simulink model "UserTire"  (Simulink 7.9)
settings: Solver=ode45  StartTime=0.0  StopTime=inf  RelTol=1e-3
PreLoadFcn:
  | UserTire_params
undefined symbols (not defined in the file): FricCoeff, Longitudinal, Side
libraries: simulink x1, CarMaker4SL x1
(part 2 of 2)

== system UserTire/CarMaker/IPG Vehicle/CarAndTrailer/Trailer/CreateBus Vhcl.Wheel.RL ==
  In1 : Inport
  Bus Creator3 : BusCreator  Inputs=14
  Demux3 : Demux  Outputs=14
  Out1 : Outport
  wires:
  Demux3/14 -> Bus Creator3/14  "Vhcl Wheel RL Trq_WhlBearing"
  Demux3/13 -> Bus Creator3/13  "Vhcl Wheel RL Trq_T2W"
  Demux3/12 -> Bus Creator3/12  "Vhcl Wheel RL SideSlip"
  Demux3/11 -> Bus Creator3/11  "Vhcl Wheel RL LongSlip"
  Demux3/10 -> Bus Creator3/10  "Vhcl Wheel RL vBelt"
  Demux3/9 -> Bus Creator3/9  "Vhcl Wheel RL Fz"
  Demux3/8 -> Bus Creator3/8  "Vhcl Wheel RL Fy"
  Demux3/7 -> Bus Creator3/7  "Vhcl Wheel RL Fx"
  Demux3/6 -> Bus Creator3/6  "Vhcl Wheel RL r_zxy z"
  Demux3/5 -> Bus Creator3/5  "Vhcl Wheel RL r_zxy y"
  Demux3/4 -> Bus Creator3/4  "Vhcl Wheel RL r_zxy x"
  Demux3/3 -> Bus Creator3/3  "Vhcl Wheel RL t z"
  Demux3/2 -> Bus Creator3/2  "Vhcl Wheel RL t y"
  In1/1 -> Demux3/1
  Bus Creator3/1 -> Out1/1
  Demux3/1 -> Bus Creator3/1  "Vhcl Wheel RL t x"

== system UserTire/CarMaker/IPG Vehicle/CarAndTrailer/Trailer/CreateBus Vhcl.Wheel.RR ==
  In1 : Inport
  Bus Creator3 : BusCreator  Inputs=14
  Demux3 : Demux  Outputs=14
  Out1 : Outport
  wires:
  Demux3/14 -> Bus Creator3/14  "Vhcl Wheel RR Trq_WhlBearing"
  Demux3/13 -> Bus Creator3/13  "Vhcl Wheel RR Trq_T2W"
  Demux3/12 -> Bus Creator3/12  "Vhcl Wheel RR SideSlip"
  Demux3/11 -> Bus Creator3/11  "Vhcl Wheel RR LongSlip"
  Demux3/10 -> Bus Creator3/10  "Vhcl Wheel RR vBelt"
  Demux3/9 -> Bus Creator3/9  "Vhcl Wheel RR Fz"
  Demux3/8 -> Bus Creator3/8  "Vhcl Wheel RR Fy"
  Demux3/7 -> Bus Creator3/7  "Vhcl Wheel RR Fx"
  Demux3/6 -> Bus Creator3/6  "Vhcl Wheel RR r_zxy z"
  Demux3/5 -> Bus Creator3/5  "Vhcl Wheel RR r_zxy y"
  Demux3/4 -> Bus Creator3/4  "Vhcl Wheel RR r_zxy x"
  Demux3/3 -> Bus Creator3/3  "Vhcl Wheel RR t z"
  Demux3/2 -> Bus Creator3/2  "Vhcl Wheel RR t y"
  In1/1 -> Demux3/1
  Bus Creator3/1 -> Out1/1
  Demux3/1 -> Bus Creator3/1  "Vhcl Wheel RR t x"

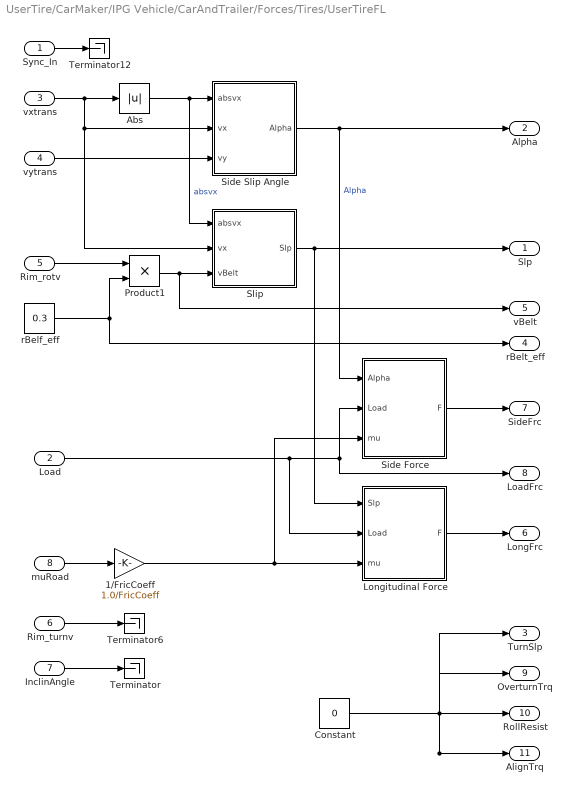
== system UserTire/CarMaker/IPG Vehicle/CarAndTrailer/Forces/Tires/UserTireFL ==
  Sync_In : Inport
  Load : Inport  Port=2
  vxtrans : Inport  Port=3
  vytrans : Inport  Port=4
  Rim_rotv : Inport  Port=5
  Rim_turnv : Inport  Port=6
  InclinAngle : Inport  Port=7
  muRoad : Inport  Port=8
  1/FricCoeff : Gain  Gain=1.0/FricCoeff  SaturateOnIntegerOverflow=on  OutDataTypeStr=Inherit: Same as input  ParamDataTypeStr=Inherit: Same as input
  Abs : Abs  SaturateOnIntegerOverflow=on
  Constant : Constant  Value=0
  Longitudinal Force : Subsystem
  Product1 : Product  Inputs=**  SaturateOnIntegerOverflow=on  InputSameDT=on  OutDataTypeStr=Inherit: Same as first input
  Side Force : Subsystem
  Side Slip Angle : Subsystem
  Slip : Subsystem
  Terminator : Terminator
  Terminator12 : Terminator
  Terminator6 : Terminator
  rBelf_eff : Constant  Value=0.3
  Slp : Outport
  Alpha : Outport  Port=2
  TurnSlp : Outport  Port=3
  rBelt_eff : Outport  Port=4
  vBelt : Outport  Port=5
  LongFrc : Outport  Port=6
  SideFrc : Outport  Port=7
  LoadFrc : Outport  Port=8
  OverturnTrq : Outport  Port=9
  RollResist : Outport  Port=10
  AlignTrq : Outport  Port=11
  wires:
  1/FricCoeff/1 -> Side Force/3(mu), Longitudinal Force/3(mu)
  muRoad/1 -> 1/FricCoeff/1
  Side Force/1(F) -> SideFrc/1
  Constant/1 -> OverturnTrq/1, RollResist/1, AlignTrq/1, TurnSlp/1
  InclinAngle/1 -> Terminator/1
  Longitudinal Force/1(F) -> LongFrc/1
  Load/1 -> LoadFrc/1, Side Force/2(Load), Longitudinal Force/2(Load)
  Slip/1(Slp) -> Slp/1, Longitudinal Force/1(Slp)
  Side Slip Angle/1(Alpha) -> Alpha/1, Side Force/1(Alpha)  "Alpha"
  Abs/1 -> Slip/1(absvx), Side Slip Angle/1(absvx)  "absvx"
  vytrans/1 -> Side Slip Angle/3(vy)
  vxtrans/1 -> Slip/2(vx), Side Slip Angle/2(vx), Abs/1
  Sync_In/1 -> Terminator12/1
  Rim_turnv/1 -> Terminator6/1
  Rim_rotv/1 -> Product1/1
  Product1/1 -> Slip/3(vBelt), vBelt/1
  rBelf_eff/1 -> Product1/2, rBelt_eff/1

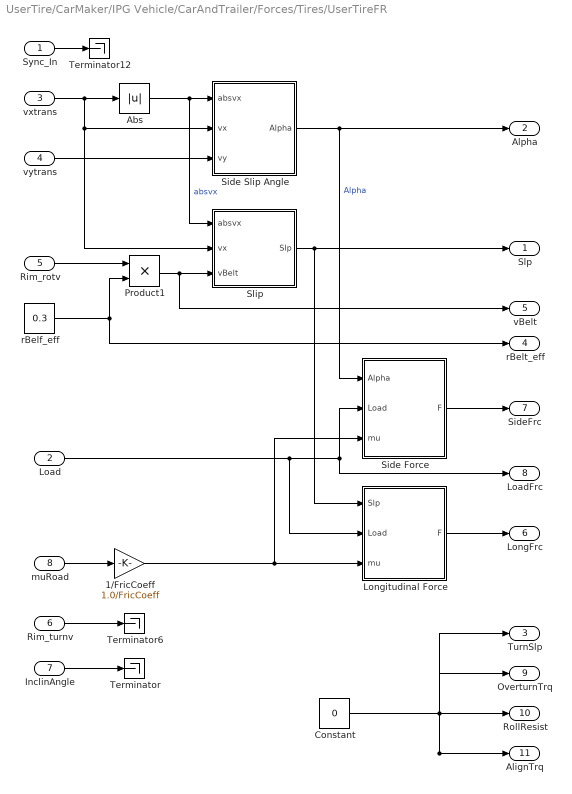
== system UserTire/CarMaker/IPG Vehicle/CarAndTrailer/Forces/Tires/UserTireFR ==
  Sync_In : Inport
  Load : Inport  Port=2
  vxtrans : Inport  Port=3
  vytrans : Inport  Port=4
  Rim_rotv : Inport  Port=5
  Rim_turnv : Inport  Port=6
  InclinAngle : Inport  Port=7
  muRoad : Inport  Port=8
  1/FricCoeff : Gain  Gain=1.0/FricCoeff  SaturateOnIntegerOverflow=on  OutDataTypeStr=Inherit: Same as input  ParamDataTypeStr=Inherit: Same as input
  Abs : Abs  SaturateOnIntegerOverflow=on
  Constant : Constant  Value=0
  Longitudinal Force : Subsystem
  Product1 : Product  Inputs=**  SaturateOnIntegerOverflow=on  InputSameDT=on  OutDataTypeStr=Inherit: Same as first input
  Side Force : Subsystem
  Side Slip Angle : Subsystem
  Slip : Subsystem
  Terminator : Terminator
  Terminator12 : Terminator
  Terminator6 : Terminator
  rBelf_eff : Constant  Value=0.3
  Slp : Outport
  Alpha : Outport  Port=2
  TurnSlp : Outport  Port=3
  rBelt_eff : Outport  Port=4
  vBelt : Outport  Port=5
  LongFrc : Outport  Port=6
  SideFrc : Outport  Port=7
  LoadFrc : Outport  Port=8
  OverturnTrq : Outport  Port=9
  RollResist : Outport  Port=10
  AlignTrq : Outport  Port=11
  wires:
  1/FricCoeff/1 -> Side Force/3(mu), Longitudinal Force/3(mu)
  muRoad/1 -> 1/FricCoeff/1
  Side Force/1(F) -> SideFrc/1
  Constant/1 -> OverturnTrq/1, RollResist/1, AlignTrq/1, TurnSlp/1
  InclinAngle/1 -> Terminator/1
  Longitudinal Force/1(F) -> LongFrc/1
  Load/1 -> LoadFrc/1, Side Force/2(Load), Longitudinal Force/2(Load)
  Slip/1(Slp) -> Slp/1, Longitudinal Force/1(Slp)
  Side Slip Angle/1(Alpha) -> Alpha/1, Side Force/1(Alpha)  "Alpha"
  Abs/1 -> Slip/1(absvx), Side Slip Angle/1(absvx)  "absvx"
  vytrans/1 -> Side Slip Angle/3(vy)
  vxtrans/1 -> Slip/2(vx), Side Slip Angle/2(vx), Abs/1
  Sync_In/1 -> Terminator12/1
  Rim_turnv/1 -> Terminator6/1
  Rim_rotv/1 -> Product1/1
  Product1/1 -> Slip/3(vBelt), vBelt/1
  rBelf_eff/1 -> Product1/2, rBelt_eff/1

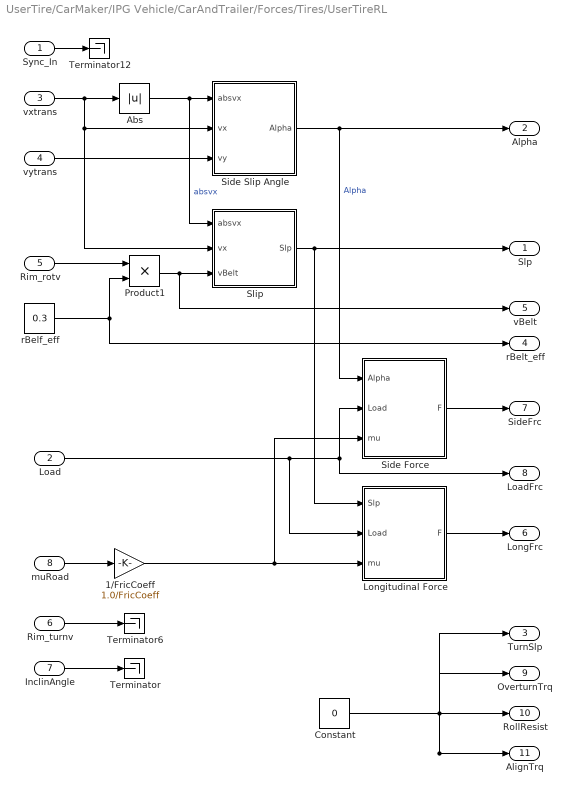
== system UserTire/CarMaker/IPG Vehicle/CarAndTrailer/Forces/Tires/UserTireRL ==
  Sync_In : Inport
  Load : Inport  Port=2
  vxtrans : Inport  Port=3
  vytrans : Inport  Port=4
  Rim_rotv : Inport  Port=5
  Rim_turnv : Inport  Port=6
  InclinAngle : Inport  Port=7
  muRoad : Inport  Port=8
  1/FricCoeff : Gain  Gain=1.0/FricCoeff  SaturateOnIntegerOverflow=on  OutDataTypeStr=Inherit: Same as input  ParamDataTypeStr=Inherit: Same as input
  Abs : Abs  SaturateOnIntegerOverflow=on
  Constant : Constant  Value=0
  Longitudinal Force : Subsystem
  Product1 : Product  Inputs=**  SaturateOnIntegerOverflow=on  InputSameDT=on  OutDataTypeStr=Inherit: Same as first input
  Side Force : Subsystem
  Side Slip Angle : Subsystem
  Slip : Subsystem
  Terminator : Terminator
  Terminator12 : Terminator
  Terminator6 : Terminator
  rBelf_eff : Constant  Value=0.3
  Slp : Outport
  Alpha : Outport  Port=2
  TurnSlp : Outport  Port=3
  rBelt_eff : Outport  Port=4
  vBelt : Outport  Port=5
  LongFrc : Outport  Port=6
  SideFrc : Outport  Port=7
  LoadFrc : Outport  Port=8
  OverturnTrq : Outport  Port=9
  RollResist : Outport  Port=10
  AlignTrq : Outport  Port=11
  wires:
  1/FricCoeff/1 -> Side Force/3(mu), Longitudinal Force/3(mu)
  muRoad/1 -> 1/FricCoeff/1
  Side Force/1(F) -> SideFrc/1
  Constant/1 -> OverturnTrq/1, RollResist/1, AlignTrq/1, TurnSlp/1
  InclinAngle/1 -> Terminator/1
  Longitudinal Force/1(F) -> LongFrc/1
  Load/1 -> LoadFrc/1, Side Force/2(Load), Longitudinal Force/2(Load)
  Slip/1(Slp) -> Slp/1, Longitudinal Force/1(Slp)
  Side Slip Angle/1(Alpha) -> Alpha/1, Side Force/1(Alpha)  "Alpha"
  Abs/1 -> Slip/1(absvx), Side Slip Angle/1(absvx)  "absvx"
  vytrans/1 -> Side Slip Angle/3(vy)
  vxtrans/1 -> Slip/2(vx), Side Slip Angle/2(vx), Abs/1
  Sync_In/1 -> Terminator12/1
  Rim_turnv/1 -> Terminator6/1
  Rim_rotv/1 -> Product1/1
  Product1/1 -> Slip/3(vBelt), vBelt/1
  rBelf_eff/1 -> Product1/2, rBelt_eff/1

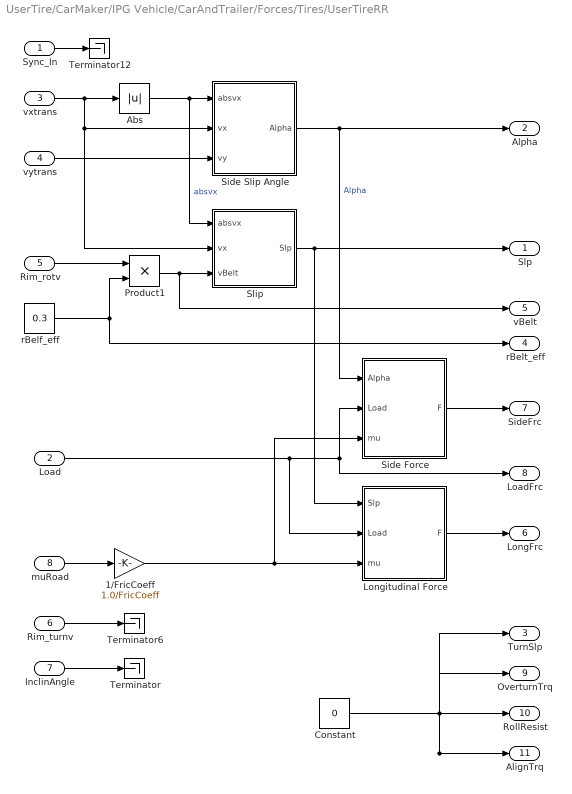
== system UserTire/CarMaker/IPG Vehicle/CarAndTrailer/Forces/Tires/UserTireRR ==
  Sync_In : Inport
  Load : Inport  Port=2
  vxtrans : Inport  Port=3
  vytrans : Inport  Port=4
  Rim_rotv : Inport  Port=5
  Rim_turnv : Inport  Port=6
  InclinAngle : Inport  Port=7
  muRoad : Inport  Port=8
  1/FricCoeff : Gain  Gain=1.0/FricCoeff  SaturateOnIntegerOverflow=on  OutDataTypeStr=Inherit: Same as input  ParamDataTypeStr=Inherit: Same as input
  Abs : Abs  SaturateOnIntegerOverflow=on
  Constant : Constant  Value=0
  Longitudinal Force : Subsystem
  Product1 : Product  Inputs=**  SaturateOnIntegerOverflow=on  InputSameDT=on  OutDataTypeStr=Inherit: Same as first input
  Side Force : Subsystem
  Side Slip Angle : Subsystem
  Slip : Subsystem
  Terminator : Terminator
  Terminator12 : Terminator
  Terminator6 : Terminator
  rBelf_eff : Constant  Value=0.3
  Slp : Outport
  Alpha : Outport  Port=2
  TurnSlp : Outport  Port=3
  rBelt_eff : Outport  Port=4
  vBelt : Outport  Port=5
  LongFrc : Outport  Port=6
  SideFrc : Outport  Port=7
  LoadFrc : Outport  Port=8
  OverturnTrq : Outport  Port=9
  RollResist : Outport  Port=10
  AlignTrq : Outport  Port=11
  wires:
  1/FricCoeff/1 -> Side Force/3(mu), Longitudinal Force/3(mu)
  muRoad/1 -> 1/FricCoeff/1
  Side Force/1(F) -> SideFrc/1
  Constant/1 -> OverturnTrq/1, RollResist/1, AlignTrq/1, TurnSlp/1
  InclinAngle/1 -> Terminator/1
  Longitudinal Force/1(F) -> LongFrc/1
  Load/1 -> LoadFrc/1, Side Force/2(Load), Longitudinal Force/2(Load)
  Slip/1(Slp) -> Slp/1, Longitudinal Force/1(Slp)
  Side Slip Angle/1(Alpha) -> Alpha/1, Side Force/1(Alpha)  "Alpha"
  Abs/1 -> Slip/1(absvx), Side Slip Angle/1(absvx)  "absvx"
  vytrans/1 -> Side Slip Angle/3(vy)
  vxtrans/1 -> Slip/2(vx), Side Slip Angle/2(vx), Abs/1
  Sync_In/1 -> Terminator12/1
  Rim_turnv/1 -> Terminator6/1
  Rim_rotv/1 -> Product1/1
  Product1/1 -> Slip/3(vBelt), vBelt/1
  rBelf_eff/1 -> Product1/2, rBelt_eff/1

== system UserTire/CarMaker/IPG Vehicle/CarAndTrailer/Forces/Tires/UserTireFL/Longitudinal Force ==
  Slp : Inport
  Load : Inport  Port=2
  mu : Inport  Port=3
  Abs2 : Abs  SaturateOnIntegerOverflow=on
  Longitudinal ForceRate : Constant  Value=Longitudinal.ForceRate
  Longitudinal FrictionRate : Constant  Value=Longitudinal.FrictionRate
  Product1 : Product  SaturateOnIntegerOverflow=on  InputSameDT=on  OutDataTypeStr=Inherit: Same as first input
  Product3 : Product  Inputs=3  SaturateOnIntegerOverflow=on  InputSameDT=on  OutDataTypeStr=Inherit: Same as first input
  Product4 : Product  SaturateOnIntegerOverflow=on  InputSameDT=on  OutDataTypeStr=Inherit: Same as first input
  Product5 : Product  SaturateOnIntegerOverflow=on  InputSameDT=on  OutDataTypeStr=Inherit: Same as first input
  Relational Operator1 : RelationalOperator  Operator=>  InputSameDT=on
  Sign : Signum
  Switch1 : Switch  Threshold=1  SaturateOnIntegerOverflow=on  InputSameDT=on
  F : Outport
  wires:
  mu/1 -> Product1/2
  Product1/1 -> F/1
  Switch1/1 -> Product1/1
  Load/1 -> Product4/1, Product3/2
  Slp/1 -> Product3/1
  Sign/1 -> Product5/1
  Product5/1 -> Switch1/1
  Relational Operator1/1 -> Switch1/2
  Abs2/1 -> Relational Operator1/1  "absF"
  Product4/1 -> Product5/2, Relational Operator1/2  "d"
  Product3/1 -> Switch1/3, Abs2/1, Sign/1  "F"
  Longitudinal FrictionRate/1 -> Product4/2
  Longitudinal ForceRate/1 -> Product3/3

== system UserTire/CarMaker/IPG Vehicle/CarAndTrailer/Forces/Tires/UserTireFL/Side Force ==
  Alpha : Inport
  Load : Inport  Port=2
  mu : Inport  Port=3
  -Side ForceAmplify : Constant  Value=-Side.ForceAmplify
  Abs2 : Abs  SaturateOnIntegerOverflow=on
  Product : Product  Inputs=3  SaturateOnIntegerOverflow=on  InputSameDT=on  OutDataTypeStr=Inherit: Same as first input
  Product3 : Product  Inputs=3  SaturateOnIntegerOverflow=on  InputSameDT=on  OutDataTypeStr=Inherit: Same as first input
  Product4 : Product  SaturateOnIntegerOverflow=on  InputSameDT=on  OutDataTypeStr=Inherit: Same as first input
  Product5 : Product  SaturateOnIntegerOverflow=on  InputSameDT=on  OutDataTypeStr=Inherit: Same as first input
  Relational Operator1 : RelationalOperator  Operator=>  InputSameDT=on
  Side ForceRate : Constant  Value=Side.ForceRate
  Side FrictionRate : Constant  Value=Side.FrictionRate
  Sign : Signum
  Switch1 : Switch  Threshold=1  SaturateOnIntegerOverflow=on  InputSameDT=on
  F : Outport
  wires:
  mu/1 -> Product/3
  -Side ForceAmplify/1 -> Product/1
  Product/1 -> F/1
  Switch1/1 -> Product/2
  Load/1 -> Product4/1, Product3/2
  Alpha/1 -> Product3/1
  Sign/1 -> Product5/1
  Product5/1 -> Switch1/1
  Relational Operator1/1 -> Switch1/2
  Abs2/1 -> Relational Operator1/1  "absF"
  Product4/1 -> Product5/2, Relational Operator1/2  "d"
  Product3/1 -> Switch1/3, Abs2/1, Sign/1  "F"
  Side FrictionRate/1 -> Product4/2
  Side ForceRate/1 -> Product3/3

== system UserTire/CarMaker/IPG Vehicle/CarAndTrailer/Forces/Tires/UserTireFL/Side Slip Angle ==
  absvx : Inport
  vx : Inport  Port=2
  vy : Inport  Port=3
  Constant6 : Constant  Value=0.25
  Constant7 : Constant  Value=0
  Relational Operator3 : RelationalOperator  Operator=>  InputSameDT=on
  Switch3 : Switch  Threshold=1  SaturateOnIntegerOverflow=on  InputSameDT=on
  Trigonometric Function1 : Trigonometry  Operator=atan2
  Alpha : Outport
  wires:
  Constant7/1 -> Switch3/3
  Trigonometric Function1/1 -> Switch3/1
  vy/1 -> Trigonometric Function1/1
  vx/1 -> Trigonometric Function1/2
  Switch3/1 -> Alpha/1
  absvx/1 -> Relational Operator3/1
  Relational Operator3/1 -> Switch3/2
  Constant6/1 -> Relational Operator3/2

== system UserTire/CarMaker/IPG Vehicle/CarAndTrailer/Forces/Tires/UserTireFL/Slip ==
  absvx : Inport
  vx : Inport  Port=2
  vBelt : Inport  Port=3
  Abs2 : Abs  SaturateOnIntegerOverflow=on
  Constant1 : Constant  Value=0
  Constant3 : Constant  Value=0
  Constant4 : Constant  Value=0.000001
  Product1 : Product  Inputs=*/  SaturateOnIntegerOverflow=on  InputSameDT=on  OutDataTypeStr=Inherit: Same as first input
  Relational Operator1 : RelationalOperator  Operator===  InputSameDT=on
  Relational Operator3 : RelationalOperator  Operator=<  InputSameDT=on
  Sum1 : Sum  Inputs=-+  SaturateOnIntegerOverflow=on  InputSameDT=on  OutDataTypeStr=Inherit: Same as first input
  Switch1 : Switch  Threshold=1  SaturateOnIntegerOverflow=on  InputSameDT=on
  Switch3 : Switch  Threshold=1  SaturateOnIntegerOverflow=on  InputSameDT=on
  Slp : Outport
  wires:
  Product1/1 -> Slp/1
  Constant4/1 -> Switch1/1
  Switch1/1 -> Product1/2  "not zero"
  Constant3/1 -> Relational Operator1/1
  Relational Operator1/1 -> Switch1/2
  vBelt/1 -> Abs2/1, Sum1/2
  absvx/1 -> Switch3/1
  vx/1 -> Sum1/1
  Switch3/1 -> Switch1/3, Relational Operator1/2  "vslp"
  Abs2/1 -> Switch3/3
  Relational Operator3/1 -> Switch3/2
  Constant1/1 -> Relational Operator3/2
  Sum1/1 -> Product1/1, Relational Operator3/1  "deltav"

== system UserTire/CarMaker/IPG Vehicle/CarAndTrailer/Forces/Tires/UserTireFR/Longitudinal Force ==
  Slp : Inport
  Load : Inport  Port=2
  mu : Inport  Port=3
  Abs2 : Abs  SaturateOnIntegerOverflow=on
  Longitudinal ForceRate : Constant  Value=Longitudinal.ForceRate
  Longitudinal FrictionRate : Constant  Value=Longitudinal.FrictionRate
  Product1 : Product  SaturateOnIntegerOverflow=on  InputSameDT=on  OutDataTypeStr=Inherit: Same as first input
  Product3 : Product  Inputs=3  SaturateOnIntegerOverflow=on  InputSameDT=on  OutDataTypeStr=Inherit: Same as first input
  Product4 : Product  SaturateOnIntegerOverflow=on  InputSameDT=on  OutDataTypeStr=Inherit: Same as first input
  Product5 : Product  SaturateOnIntegerOverflow=on  InputSameDT=on  OutDataTypeStr=Inherit: Same as first input
  Relational Operator1 : RelationalOperator  Operator=>  InputSameDT=on
  Sign : Signum
  Switch1 : Switch  Threshold=1  SaturateOnIntegerOverflow=on  InputSameDT=on
  F : Outport
  wires:
  mu/1 -> Product1/2
  Product1/1 -> F/1
  Switch1/1 -> Product1/1
  Load/1 -> Product4/1, Product3/2
  Slp/1 -> Product3/1
  Sign/1 -> Product5/1
  Product5/1 -> Switch1/1
  Relational Operator1/1 -> Switch1/2
  Abs2/1 -> Relational Operator1/1  "absF"
  Product4/1 -> Product5/2, Relational Operator1/2  "d"
  Product3/1 -> Switch1/3, Abs2/1, Sign/1  "F"
  Longitudinal FrictionRate/1 -> Product4/2
  Longitudinal ForceRate/1 -> Product3/3

== system UserTire/CarMaker/IPG Vehicle/CarAndTrailer/Forces/Tires/UserTireFR/Side Force ==
  Alpha : Inport
  Load : Inport  Port=2
  mu : Inport  Port=3
  -Side ForceAmplify : Constant  Value=-Side.ForceAmplify
  Abs2 : Abs  SaturateOnIntegerOverflow=on
  Product : Product  Inputs=3  SaturateOnIntegerOverflow=on  InputSameDT=on  OutDataTypeStr=Inherit: Same as first input
  Product3 : Product  Inputs=3  SaturateOnIntegerOverflow=on  InputSameDT=on  OutDataTypeStr=Inherit: Same as first input
  Product4 : Product  SaturateOnIntegerOverflow=on  InputSameDT=on  OutDataTypeStr=Inherit: Same as first input
  Product5 : Product  SaturateOnIntegerOverflow=on  InputSameDT=on  OutDataTypeStr=Inherit: Same as first input
  Relational Operator1 : RelationalOperator  Operator=>  InputSameDT=on
  Side ForceRate : Constant  Value=Side.ForceRate
  Side FrictionRate : Constant  Value=Side.FrictionRate
  Sign : Signum
  Switch1 : Switch  Threshold=1  SaturateOnIntegerOverflow=on  InputSameDT=on
  F : Outport
  wires:
  mu/1 -> Product/3
  -Side ForceAmplify/1 -> Product/1
  Product/1 -> F/1
  Switch1/1 -> Product/2
  Load/1 -> Product4/1, Product3/2
  Alpha/1 -> Product3/1
  Sign/1 -> Product5/1
  Product5/1 -> Switch1/1
  Relational Operator1/1 -> Switch1/2
  Abs2/1 -> Relational Operator1/1  "absF"
  Product4/1 -> Product5/2, Relational Operator1/2  "d"
  Product3/1 -> Switch1/3, Abs2/1, Sign/1  "F"
  Side FrictionRate/1 -> Product4/2
  Side ForceRate/1 -> Product3/3

== system UserTire/CarMaker/IPG Vehicle/CarAndTrailer/Forces/Tires/UserTireFR/Side Slip Angle ==
  absvx : Inport
  vx : Inport  Port=2
  vy : Inport  Port=3
  Constant6 : Constant  Value=0.25
  Constant7 : Constant  Value=0
  Relational Operator3 : RelationalOperator  Operator=>  InputSameDT=on
  Switch3 : Switch  Threshold=1  SaturateOnIntegerOverflow=on  InputSameDT=on
  Trigonometric Function1 : Trigonometry  Operator=atan2
  Alpha : Outport
  wires:
  Constant7/1 -> Switch3/3
  Trigonometric Function1/1 -> Switch3/1
  vy/1 -> Trigonometric Function1/1
  vx/1 -> Trigonometric Function1/2
  Switch3/1 -> Alpha/1
  absvx/1 -> Relational Operator3/1
  Relational Operator3/1 -> Switch3/2
  Constant6/1 -> Relational Operator3/2

== system UserTire/CarMaker/IPG Vehicle/CarAndTrailer/Forces/Tires/UserTireFR/Slip ==
  absvx : Inport
  vx : Inport  Port=2
  vBelt : Inport  Port=3
  Abs2 : Abs  SaturateOnIntegerOverflow=on
  Constant1 : Constant  Value=0
  Constant3 : Constant  Value=0
  Constant4 : Constant  Value=0.000001
  Product1 : Product  Inputs=*/  SaturateOnIntegerOverflow=on  InputSameDT=on  OutDataTypeStr=Inherit: Same as first input
  Relational Operator1 : RelationalOperator  Operator===  InputSameDT=on
  Relational Operator3 : RelationalOperator  Operator=<  InputSameDT=on
  Sum1 : Sum  Inputs=-+  SaturateOnIntegerOverflow=on  InputSameDT=on  OutDataTypeStr=Inherit: Same as first input
  Switch1 : Switch  Threshold=1  SaturateOnIntegerOverflow=on  InputSameDT=on
  Switch3 : Switch  Threshold=1  SaturateOnIntegerOverflow=on  InputSameDT=on
  Slp : Outport
  wires:
  Product1/1 -> Slp/1
  Constant4/1 -> Switch1/1
  Switch1/1 -> Product1/2  "not zero"
  Constant3/1 -> Relational Operator1/1
  Relational Operator1/1 -> Switch1/2
  vBelt/1 -> Abs2/1, Sum1/2
  absvx/1 -> Switch3/1
  vx/1 -> Sum1/1
  Switch3/1 -> Switch1/3, Relational Operator1/2  "vslp"
  Abs2/1 -> Switch3/3
  Relational Operator3/1 -> Switch3/2
  Constant1/1 -> Relational Operator3/2
  Sum1/1 -> Product1/1, Relational Operator3/1  "deltav"

== system UserTire/CarMaker/IPG Vehicle/CarAndTrailer/Forces/Tires/UserTireRL/Longitudinal Force ==
  Slp : Inport
  Load : Inport  Port=2
  mu : Inport  Port=3
  Abs2 : Abs  SaturateOnIntegerOverflow=on
  Longitudinal ForceRate : Constant  Value=Longitudinal.ForceRate
  Longitudinal FrictionRate : Constant  Value=Longitudinal.FrictionRate
  Product1 : Product  SaturateOnIntegerOverflow=on  InputSameDT=on  OutDataTypeStr=Inherit: Same as first input
  Product3 : Product  Inputs=3  SaturateOnIntegerOverflow=on  InputSameDT=on  OutDataTypeStr=Inherit: Same as first input
  Product4 : Product  SaturateOnIntegerOverflow=on  InputSameDT=on  OutDataTypeStr=Inherit: Same as first input
  Product5 : Product  SaturateOnIntegerOverflow=on  InputSameDT=on  OutDataTypeStr=Inherit: Same as first input
  Relational Operator1 : RelationalOperator  Operator=>  InputSameDT=on
  Sign : Signum
  Switch1 : Switch  Threshold=1  SaturateOnIntegerOverflow=on  InputSameDT=on
  F : Outport
  wires:
  mu/1 -> Product1/2
  Product1/1 -> F/1
  Switch1/1 -> Product1/1
  Load/1 -> Product4/1, Product3/2
  Slp/1 -> Product3/1
  Sign/1 -> Product5/1
  Product5/1 -> Switch1/1
  Relational Operator1/1 -> Switch1/2
  Abs2/1 -> Relational Operator1/1  "absF"
  Product4/1 -> Product5/2, Relational Operator1/2  "d"
  Product3/1 -> Switch1/3, Abs2/1, Sign/1  "F"
  Longitudinal FrictionRate/1 -> Product4/2
  Longitudinal ForceRate/1 -> Product3/3

== system UserTire/CarMaker/IPG Vehicle/CarAndTrailer/Forces/Tires/UserTireRL/Side Force ==
  Alpha : Inport
  Load : Inport  Port=2
  mu : Inport  Port=3
  -Side ForceAmplify : Constant  Value=-Side.ForceAmplify
  Abs2 : Abs  SaturateOnIntegerOverflow=on
  Product : Product  Inputs=3  SaturateOnIntegerOverflow=on  InputSameDT=on  OutDataTypeStr=Inherit: Same as first input
  Product3 : Product  Inputs=3  SaturateOnIntegerOverflow=on  InputSameDT=on  OutDataTypeStr=Inherit: Same as first input
  Product4 : Product  SaturateOnIntegerOverflow=on  InputSameDT=on  OutDataTypeStr=Inherit: Same as first input
  Product5 : Product  SaturateOnIntegerOverflow=on  InputSameDT=on  OutDataTypeStr=Inherit: Same as first input
  Relational Operator1 : RelationalOperator  Operator=>  InputSameDT=on
  Side ForceRate : Constant  Value=Side.ForceRate
  Side FrictionRate : Constant  Value=Side.FrictionRate
  Sign : Signum
  Switch1 : Switch  Threshold=1  SaturateOnIntegerOverflow=on  InputSameDT=on
  F : Outport
  wires:
  mu/1 -> Product/3
  -Side ForceAmplify/1 -> Product/1
  Product/1 -> F/1
  Switch1/1 -> Product/2
  Load/1 -> Product4/1, Product3/2
  Alpha/1 -> Product3/1
  Sign/1 -> Product5/1
  Product5/1 -> Switch1/1
  Relational Operator1/1 -> Switch1/2
  Abs2/1 -> Relational Operator1/1  "absF"
  Product4/1 -> Product5/2, Relational Operator1/2  "d"
  Product3/1 -> Switch1/3, Abs2/1, Sign/1  "F"
  Side FrictionRate/1 -> Product4/2
  Side ForceRate/1 -> Product3/3

== system UserTire/CarMaker/IPG Vehicle/CarAndTrailer/Forces/Tires/UserTireRL/Side Slip Angle ==
  absvx : Inport
  vx : Inport  Port=2
  vy : Inport  Port=3
  Constant6 : Constant  Value=0.25
  Constant7 : Constant  Value=0
  Relational Operator3 : RelationalOperator  Operator=>  InputSameDT=on
  Switch3 : Switch  Threshold=1  SaturateOnIntegerOverflow=on  InputSameDT=on
  Trigonometric Function1 : Trigonometry  Operator=atan2
  Alpha : Outport
  wires:
  Constant7/1 -> Switch3/3
  Trigonometric Function1/1 -> Switch3/1
  vy/1 -> Trigonometric Function1/1
  vx/1 -> Trigonometric Function1/2
  Switch3/1 -> Alpha/1
  absvx/1 -> Relational Operator3/1
  Relational Operator3/1 -> Switch3/2
  Constant6/1 -> Relational Operator3/2

== system UserTire/CarMaker/IPG Vehicle/CarAndTrailer/Forces/Tires/UserTireRL/Slip ==
  absvx : Inport
  vx : Inport  Port=2
  vBelt : Inport  Port=3
  Abs2 : Abs  SaturateOnIntegerOverflow=on
  Constant1 : Constant  Value=0
  Constant3 : Constant  Value=0
  Constant4 : Constant  Value=0.000001
  Product1 : Product  Inputs=*/  SaturateOnIntegerOverflow=on  InputSameDT=on  OutDataTypeStr=Inherit: Same as first input
  Relational Operator1 : RelationalOperator  Operator===  InputSameDT=on
  Relational Operator3 : RelationalOperator  Operator=<  InputSameDT=on
  Sum1 : Sum  Inputs=-+  SaturateOnIntegerOverflow=on  InputSameDT=on  OutDataTypeStr=Inherit: Same as first input
  Switch1 : Switch  Threshold=1  SaturateOnIntegerOverflow=on  InputSameDT=on
  Switch3 : Switch  Threshold=1  SaturateOnIntegerOverflow=on  InputSameDT=on
  Slp : Outport
  wires:
  Product1/1 -> Slp/1
  Constant4/1 -> Switch1/1
  Switch1/1 -> Product1/2  "not zero"
  Constant3/1 -> Relational Operator1/1
  Relational Operator1/1 -> Switch1/2
  vBelt/1 -> Abs2/1, Sum1/2
  absvx/1 -> Switch3/1
  vx/1 -> Sum1/1
  Switch3/1 -> Switch1/3, Relational Operator1/2  "vslp"
  Abs2/1 -> Switch3/3
  Relational Operator3/1 -> Switch3/2
  Constant1/1 -> Relational Operator3/2
  Sum1/1 -> Product1/1, Relational Operator3/1  "deltav"

== system UserTire/CarMaker/IPG Vehicle/CarAndTrailer/Forces/Tires/UserTireRR/Longitudinal Force ==
  Slp : Inport
  Load : Inport  Port=2
  mu : Inport  Port=3
  Abs2 : Abs  SaturateOnIntegerOverflow=on
  Longitudinal ForceRate : Constant  Value=Longitudinal.ForceRate
  Longitudinal FrictionRate : Constant  Value=Longitudinal.FrictionRate
  Product1 : Product  SaturateOnIntegerOverflow=on  InputSameDT=on  OutDataTypeStr=Inherit: Same as first input
  Product3 : Product  Inputs=3  SaturateOnIntegerOverflow=on  InputSameDT=on  OutDataTypeStr=Inherit: Same as first input
  Product4 : Product  SaturateOnIntegerOverflow=on  InputSameDT=on  OutDataTypeStr=Inherit: Same as first input
  Product5 : Product  SaturateOnIntegerOverflow=on  InputSameDT=on  OutDataTypeStr=Inherit: Same as first input
  Relational Operator1 : RelationalOperator  Operator=>  InputSameDT=on
  Sign : Signum
  Switch1 : Switch  Threshold=1  SaturateOnIntegerOverflow=on  InputSameDT=on
  F : Outport
  wires:
  mu/1 -> Product1/2
  Product1/1 -> F/1
  Switch1/1 -> Product1/1
  Load/1 -> Product4/1, Product3/2
  Slp/1 -> Product3/1
  Sign/1 -> Product5/1
  Product5/1 -> Switch1/1
  Relational Operator1/1 -> Switch1/2
  Abs2/1 -> Relational Operator1/1  "absF"
  Product4/1 -> Product5/2, Relational Operator1/2  "d"
  Product3/1 -> Switch1/3, Abs2/1, Sign/1  "F"
  Longitudinal FrictionRate/1 -> Product4/2
  Longitudinal ForceRate/1 -> Product3/3

== system UserTire/CarMaker/IPG Vehicle/CarAndTrailer/Forces/Tires/UserTireRR/Side Force ==
  Alpha : Inport
  Load : Inport  Port=2
  mu : Inport  Port=3
  -Side ForceAmplify : Constant  Value=-Side.ForceAmplify
  Abs2 : Abs  SaturateOnIntegerOverflow=on
  Product : Product  Inputs=3  SaturateOnIntegerOverflow=on  InputSameDT=on  OutDataTypeStr=Inherit: Same as first input
  Product3 : Product  Inputs=3  SaturateOnIntegerOverflow=on  InputSameDT=on  OutDataTypeStr=Inherit: Same as first input
  Product4 : Product  SaturateOnIntegerOverflow=on  InputSameDT=on  OutDataTypeStr=Inherit: Same as first input
  Product5 : Product  SaturateOnIntegerOverflow=on  InputSameDT=on  OutDataTypeStr=Inherit: Same as first input
  Relational Operator1 : RelationalOperator  Operator=>  InputSameDT=on
  Side ForceRate : Constant  Value=Side.ForceRate
  Side FrictionRate : Constant  Value=Side.FrictionRate
  Sign : Signum
  Switch1 : Switch  Threshold=1  SaturateOnIntegerOverflow=on  InputSameDT=on
  F : Outport
  wires:
  mu/1 -> Product/3
  -Side ForceAmplify/1 -> Product/1
  Product/1 -> F/1
  Switch1/1 -> Product/2
  Load/1 -> Product4/1, Product3/2
  Alpha/1 -> Product3/1
  Sign/1 -> Product5/1
  Product5/1 -> Switch1/1
  Relational Operator1/1 -> Switch1/2
  Abs2/1 -> Relational Operator1/1  "absF"
  Product4/1 -> Product5/2, Relational Operator1/2  "d"
  Product3/1 -> Switch1/3, Abs2/1, Sign/1  "F"
  Side FrictionRate/1 -> Product4/2
  Side ForceRate/1 -> Product3/3

== system UserTire/CarMaker/IPG Vehicle/CarAndTrailer/Forces/Tires/UserTireRR/Side Slip Angle ==
  absvx : Inport
  vx : Inport  Port=2
  vy : Inport  Port=3
  Constant6 : Constant  Value=0.25
  Constant7 : Constant  Value=0
  Relational Operator3 : RelationalOperator  Operator=>  InputSameDT=on
  Switch3 : Switch  Threshold=1  SaturateOnIntegerOverflow=on  InputSameDT=on
  Trigonometric Function1 : Trigonometry  Operator=atan2
  Alpha : Outport
  wires:
  Constant7/1 -> Switch3/3
  Trigonometric Function1/1 -> Switch3/1
  vy/1 -> Trigonometric Function1/1
  vx/1 -> Trigonometric Function1/2
  Switch3/1 -> Alpha/1
  absvx/1 -> Relational Operator3/1
  Relational Operator3/1 -> Switch3/2
  Constant6/1 -> Relational Operator3/2

== system UserTire/CarMaker/IPG Vehicle/CarAndTrailer/Forces/Tires/UserTireRR/Slip ==
  absvx : Inport
  vx : Inport  Port=2
  vBelt : Inport  Port=3
  Abs2 : Abs  SaturateOnIntegerOverflow=on
  Constant1 : Constant  Value=0
  Constant3 : Constant  Value=0
  Constant4 : Constant  Value=0.000001
  Product1 : Product  Inputs=*/  SaturateOnIntegerOverflow=on  InputSameDT=on  OutDataTypeStr=Inherit: Same as first input
  Relational Operator1 : RelationalOperator  Operator===  InputSameDT=on
  Relational Operator3 : RelationalOperator  Operator=<  InputSameDT=on
  Sum1 : Sum  Inputs=-+  SaturateOnIntegerOverflow=on  InputSameDT=on  OutDataTypeStr=Inherit: Same as first input
  Switch1 : Switch  Threshold=1  SaturateOnIntegerOverflow=on  InputSameDT=on
  Switch3 : Switch  Threshold=1  SaturateOnIntegerOverflow=on  InputSameDT=on
  Slp : Outport
  wires:
  Product1/1 -> Slp/1
  Constant4/1 -> Switch1/1
  Switch1/1 -> Product1/2  "not zero"
  Constant3/1 -> Relational Operator1/1
  Relational Operator1/1 -> Switch1/2
  vBelt/1 -> Abs2/1, Sum1/2
  absvx/1 -> Switch3/1
  vx/1 -> Sum1/1
  Switch3/1 -> Switch1/3, Relational Operator1/2  "vslp"
  Abs2/1 -> Switch3/3
  Relational Operator3/1 -> Switch3/2
  Constant1/1 -> Relational Operator3/2
  Sum1/1 -> Product1/1, Relational Operator3/1  "deltav"
